simulink model "Controls_Simulation"  (R2022b)
settings: Solver=VariableStepAuto  StartTime=0.0  StopTime=20  RelTol=1e-3
libraries: slpidlib x5
settings Model: Creator=VIGNESH  LastModifiedBy=sandi

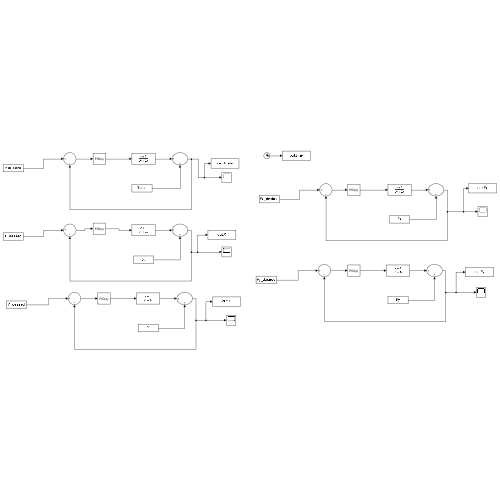
[thumbnail: Simulink's stored preview of the top-level diagram]
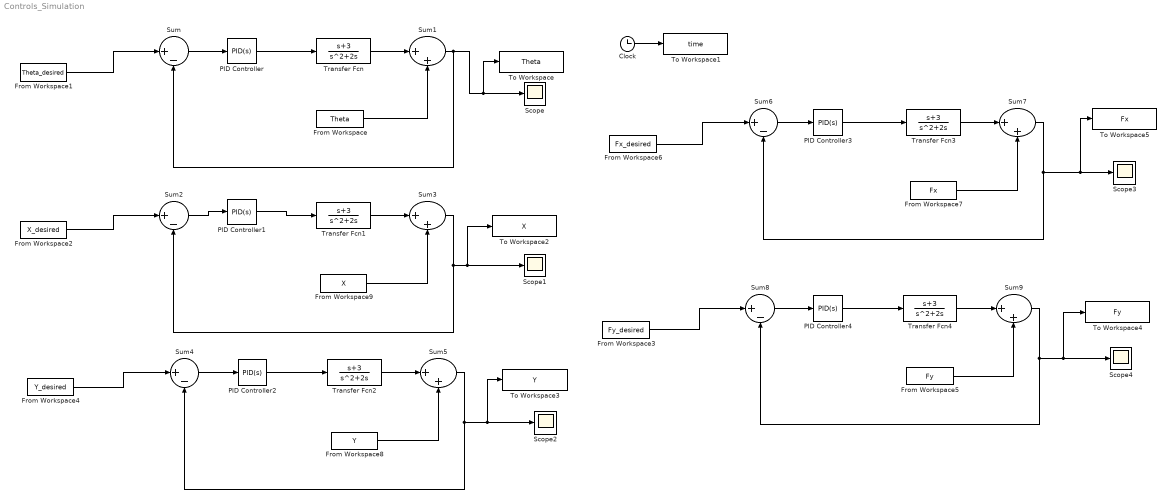
== system Controls_Simulation ==
  Clock : Clock
  From Workspace : FromWorkspace  VariableName=Theta
  From Workspace1 : FromWorkspace  VariableName=Theta_desired
  From Workspace2 : FromWorkspace  VariableName=X_desired
  From Workspace3 : FromWorkspace  VariableName=Fy_desired
  From Workspace4 : FromWorkspace  VariableName=Y_desired
  From Workspace5 : FromWorkspace  VariableName=Fy
  From Workspace6 : FromWorkspace  VariableName=Fx_desired
  From Workspace7 : FromWorkspace  VariableName=Fx
  From Workspace8 : FromWorkspace  VariableName=Y
  From Workspace9 : FromWorkspace  VariableName=X
  PID Controller{,1..4} (5 alike) : slpidlib/PID Controller  Controller=PID  Form=Parallel  TimeDomain=Continuous-time  UseExternalTs=off  SampleTime=-1  IntegratorMethod=Forward Euler  FilterMethod=Forward Euler  ControllerParametersSource=internal  P=0.842712233998587  I=0  UseKiTs=off  D=-0.066821402381307  N=0.0312  UseFilter=on  TunerSelectOption=Transfer Function Based (PID Tuner App)  InitialConditionSource=internal  InitialConditionForIntegrator=0  InitialConditionForFilter=0  DifferentiatorICPrevScaledInput=0  ExternalReset=none  TrackingMode=off  Kt=1  LimitOutput=off  SatLimitsSource=internal  UpperSaturationLimit=inf  LowerSaturationLimit=-inf  LinearizeAsGain=on  AntiWindupMode=none  Kb=1  LimitIntegrator=off  UpperIntegratorSaturationLimit=inf  LowerIntegratorSaturationLimit=-inf  POutMin=[]  POutMax=[]  IOutMin=[]  IOutMax=[]  DOutMin=[]  DOutMax=[]  NOutMin=[]  NOutMax=[]  SumOutMin=[]  SumOutMax=[]  SaturationOutMin=[]  SaturationOutMax=[]  PParamMin=[]  PParamMax=[]  IParamMin=[]  IParamMax=[]  DParamMin=[]  DParamMax=[]  NParamMin=[]  NParamMax=[]  KbParamMin=[]  KbParamMax=[]  KtParamMin=[]  KtParamMax=[]  KbOutMin=[]  KbOutMax=[]  KtOutMin=[]  KtOutMax=[]  IntegratorOutMin=[]  IntegratorOutMax=[]  FilterOutMin=[]  FilterOutMax=[]  SumI1OutMin=[]  SumI1OutMax=[]  SumI2OutMin=[]  SumI2OutMax=[]  SumI3OutMin=[]  SumI3OutMax=[]  SumI4OutMin=[]  SumI4OutMax=[]  SumDOutMin=[]  SumDOutMax=[]  DifferentiatorOutMin=[]  DifferentiatorOutMax=[]  FilterDiffOutCoefMin=[]  FilterDiffOutCoefMax=[]  ReciprocalOutMin=[]  ReciprocalOutMax=[]  SumDenOutMin=[]  SumDenOutMax=[]  SumNumOutMin=[]  SumNumOutMax=[]  DivideOutMin=[]  DivideOutMax=[]  UdiffTsProdOutMin=[]  UdiffTsProdOutMax=[]  NTsProdOutMin=[]  NTsProdOutMax=[]  UintegralTsProdOutMin=[]  UintegralTsProdOutMax=[]  UngainTsProdOutMin=[]  UngainTsProdOutMax=[]  ClampingZeroOutDataTypeStr=Inherit: Inherit via back propagation  ClampingZeroOutMin=[]  ClampingZeroOutMax=[]  FilterDenConstantOutDataTypeStr=Inherit: Inherit via back propagation  FilterDenConstantOutMin=[]  FilterDenConstantOutMax=[]  PCopyOutDataTypeStr=Inherit: Inherit via back propagation  PCopyOutMin=[]  PCopyOutMax=[]  NCopyOutDataTypeStr=Inherit: Inherit via back propagation  NCopyOutMin=[]  NCopyOutMax=[]  IntegratorContinuousStateAttributes=''  IntegratorStateMustResolveToSignalObject=off  IntegratorRTWStateStorageClass=Auto  FilterContinuousStateAttributes=''  FilterStateMustResolveToSignalObject=off  FilterRTWStateStorageClass=Auto  ParallelPVariant=InternalParameters  IdealPVariant=Disabled  IVariant=InternalParameters  DVariant=InternalParameters  IntegratorVariant=Continuous  SatVariant=Disabled  AWVariant=Passthrough  PCopyVariant=Disabled  TRVariant=Disabled  FdbkBlocksVariant=Forward  IdealPFdbkVariant=Disabled  SatFdbkVariant=Disabled  DerivativeFilterVariant=ContFilter  NVariant=InternalParameters  NCopyVariant=Disabled  FilterICVariant=InternalICsFilter  IntegratorICVariant=InternalICs  ExternalResetVariant=Disabled  TRSumVariant=Passthrough  SumFdbkVariant=Disabled  SumVariant=Sum_PID  TsampFilterVariant=InternalTs  TsampNgainVariant=Passthrough  TsampIntegralVariant=Passthrough  ExternalSaturationOutDataTypeStr=Inherit: Same as second input
  Scope{,1..4} (5 alike) : Scope
  Sum{,2,4,6,8} (5 alike) : Sum  Inputs=|+-
  Sum{1,3,5,7,9} (5 alike) : Sum  Inputs=|++
  To Workspace : ToWorkspace  VariableName=Theta  SampleTime=-1
  To Workspace1 : ToWorkspace  VariableName=time  SampleTime=-1
  To Workspace2 : ToWorkspace  VariableName=X  SampleTime=-1
  To Workspace3 : ToWorkspace  VariableName=Y  SampleTime=-1
  To Workspace4 : ToWorkspace  VariableName=Fy  SampleTime=-1
  To Workspace5 : ToWorkspace  VariableName=Fx  SampleTime=-1
  Transfer Fcn{,1..4} (5 alike) : TransferFcn  Numerator=[1 3]  Denominator=[1 2 0]
  wires:
  Sum/1 -> PID Controller/1
  PID Controller/1 -> Transfer Fcn/1
  Transfer Fcn/1 -> Sum1/1
  Sum1/1 -> Sum/2, To Workspace/1, Scope/1
  From Workspace1/1 -> Sum/1
  From Workspace/1 -> Sum1/2
  From Workspace9/1 -> Sum3/2
  From Workspace2/1 -> Sum2/1
  Sum3/1 -> Sum2/2, To Workspace2/1, Scope1/1
  Transfer Fcn1/1 -> Sum3/1
  PID Controller1/1 -> Transfer Fcn1/1
  Sum2/1 -> PID Controller1/1
  PID Controller2/1 -> Transfer Fcn2/1
  Sum4/1 -> PID Controller2/1
  From Workspace4/1 -> Sum4/1
  Transfer Fcn2/1 -> Sum5/1
  Sum5/1 -> Sum4/2, To Workspace3/1, Scope2/1
  From Workspace8/1 -> Sum5/2
  From Workspace6/1 -> Sum6/1
  Sum6/1 -> PID Controller3/1
  From Workspace7/1 -> Sum7/2
  PID Controller3/1 -> Transfer Fcn3/1
  Transfer Fcn3/1 -> Sum7/1
  Sum7/1 -> Sum6/2, To Workspace5/1, Scope3/1
  From Workspace3/1 -> Sum8/1
  Sum8/1 -> PID Controller4/1
  From Workspace5/1 -> Sum9/2
  Sum9/1 -> Sum8/2, To Workspace4/1, Scope4/1
  Transfer Fcn4/1 -> Sum9/1
  PID Controller4/1 -> Transfer Fcn4/1
  Clock/1 -> To Workspace1/1
